simulink model "QuadSimulationSineSweepVrep"  (R2013b)
settings: Solver=ode1  StartTime=0  StopTime=10  FixedStep=0.01  MaxStep=0.06  RelTol=1e-3
model workspace (MAT data in the model file):
  Sig = Simulink.Signal
  Sig.DataType = 'auto'
  Sig.Dimensions = -1
  Sig.DimensionsMode = 'auto'
  Sig.Complexity = 'auto'
  Sig.SampleTime = -1
  Sig.SamplingMode = 'auto'
values from neighbouring files (symbols this model uses):
  IC = struct('P',(P),'Q',(Q),'R',(R),'Phi',(Phi),'The',(The),'Psi',(Psi),     'U',(U),'V',(V),'W',(W),'X',(X),'Y',(Y),'Z',(Z),'w1',(w1),'w2',(w2),'w3',(w3),'w4',(w4))    [ICgen.m]    (also in quadcopterDynamicsSFunction.m = block.DialogPrm(2).Data; quadcopterDynamicsSFunctionVrepV4.m = block.DialogPrm(2).Data; quadcopterDynamicsSFunctionVrepV5.m = block.DialogPrm(2).Data; quadcopterDynamicsSFunctionVrepV6.m = block.DialogPrm(2).Data)
  quadModel = struct('g',(g),'d',(d),'mass',(mass),'ct',(ct),'cq',(cq),     'Jx',(Jx),'Jy',(Jy),'Jz',(Jz),'Jm',(Jm),'Jb',(Jb),'Jbinv',(Jbinv),'dctcq',(dctcq),     'motor_m',(motor_m),'motor_dm',(motor_dm),'motor_h',(motor_h),'motor_r',(motor_r),     'ESC_m',(ESC_m),'ESC_a',(ESC_a),'ESC_b',(ESC_b),'ESC_ds',(ESC_ds),     'HUB_m',(HUB_m),'HUB_r',(HUB_r),'HUB_H',(HUB_H),     'arms_m',(arms_m),'arms_r',(arms_r),'arm ...(+111 chars)    [ModelGen.m]
  uart_up_p_10 = 0.9    [InitOnboardMatlab.m]
  uart_up_p_11 = 0.5    [InitOnboardMatlab.m]
  uart_up_p_12 = 0.1    [InitOnboardMatlab.m]
  uart_up_p_13 = 10    [InitOnboardMatlab.m]
  uart_up_p_14 = 50    [InitOnboardMatlab.m]
undefined symbols (not defined in the file or in its folder): DiscIntNeverNeededParam
libraries: simulink x6
Description:
  | This is a configurable quadcopter simulation.
  | This Simulink model demonstates attitude control.
  | 
  | Additional quadcopter modeling and simulation materials available at:
  | github.com/dch33/Quad-Sim
  | 
  | Copyright (C) 2014 D. Hartman, K. Landis, S. Moreno, J. Kim, M. Mehrer
  | 
  | License:
  |     This program is free software: you can redistribute it and/or modify
  |     it under the terms of the GNU LESSER GENERAL PUBLIC LICENSE as published by
  |     the Free Software Foundation, either version 3 of the License, or
  |     (at your option) any later version.
  | 
  |     This program is distributed in the hope that it will be useful,
  |     but WITHOUT ANY WARRANTY; without even the implied warranty of
  |     MERCHANTABILITY or FITNESS FOR A PARTICULAR PURPOSE.  See the
  |     GNU General Public License for more details.
  | 
  |     You should have received a copy of the GNU LESSER GENERAL PUBLIC LICENSE
  |     along with this program.  If not, see <http://www.gnu.org/licenses/>.
settings Model: ModifiedComment=Javid -- Thu Feb 04 15:27:35 2016 -- Version 1.32  Creator=David Hartman  LastModifiedBy=Javid
settings Model: ModifiedHistory=|
  | Javid -- Thu Feb 04 15:27:35 2016 -- Version 1.32
  | 
  | 
  | Javid -- Thu Feb 04 15:12:08 2016 -- Version 1.31
  | 
  | 
  | Javid -- Thu Feb 04 09:55:33 2016 -- Version 1.30
  | 
  | 
  | Javid -- Wed Feb 03 15:49:53 2016 -- Version 1.29
  | 
  | 
  | Javid -- Wed Feb 03 15:48:00 2016 -- Version 1.28
  | 
  | 
  | Javid -- Wed Feb 03 13:44:15 2016 -- Version 1.27
  | 
  | 
  | Javid -- Wed Feb 03 12:44:20 2016 -- Version 1.26
  | 
  | 
  | Javid -- Wed Feb 03 12:44:00 2016 -- Version 1.25
  | 
  | 
  | Javid -- Wed Feb 03 12:37:08 2016 -- Version 1.24
  | 
  | 
  | Javid -- Wed Feb 03 09:45:40 2016 -- Version 1.23
  | 
  | 
  | Javid -- Wed Feb 03 09:38:53 2016 -- Version 1.22
  | 
  | 
  | Javid -- Wed Feb 03 09:38:40 2016 -- Version 1.21
  | 
  | 
  | Javid -- Sat Dec 12 20:58:12 2015 -- Version 1.20
  | 
  | 
  | Javid -- Sun Nov 29 22:14:37 2015 -- Version 1.19
  | 
  | 
  | Javid -- Sun Nov 29 17:38:57 2015 -- Version 1.18
  | 
  | 
  | Javid -- Sun Nov 29 17:36:33 2015 -- Version 1.17
  | 
  | 
  | Javid -- Sun Nov 29 17:16:16 2015 -- Version 1.16
  | 
  | 
  | Javid -- Sun Nov 29 16:59:28 2015 -- Version 1.15
  | 
  | 
  | Javid -- Sun Nov 29 16:48:02 2015 -- Version 1.14
  | 
  | 
  | Javid -- Sun Nov 29 16:04:55 2015 -- Version 1.13
  | 
  | 
  | Javid -- Sat Oct 31 23:55:35 2015 -- Version 1.12
  | 
  | 
  | Javid -- Sat Oct 31 20:30:45 2015 -- Version 1.11
  | 
  | 
  | Cavid -- Mon Oct 19 16:53:56 2015 -- Version 1.10
  | 
  | 
  | Cavid -- Mon Oct 19 11:55:21 2015 -- Version 1.9
  | 
  | 
  | Cavid -- Mon Oct 19 11:50:10 2015 -- Version 1.8
  | 
  | 
  | Cavid -- Mon Oct 19 11:48:50 2015 -- Version 1.7
  | 
  | 
  | Cavid -- Mon Oct 19 11:27:32 2015 -- Version 1.6
  | 
  | 
  | davidhartman -- Fri Jun 06 23:19:51 2014 -- Version 1.5
  | 
  | 
  | davidhartman -- Fri Jun 06 22:53:10 2014 -- Version 1.3
settings SolverCC: AutoInsertRateTranBlk=on
settings DataIOCC: LimitDataPoints=off  SignalLogging=off
settings OptimizationCC: InlineParams=on
settings DebuggingCC: UniqueDataStoreMsg=warning  StateNameClashWarn=warning  StrictBusMsg=WarnOnBusTreatedAsVector

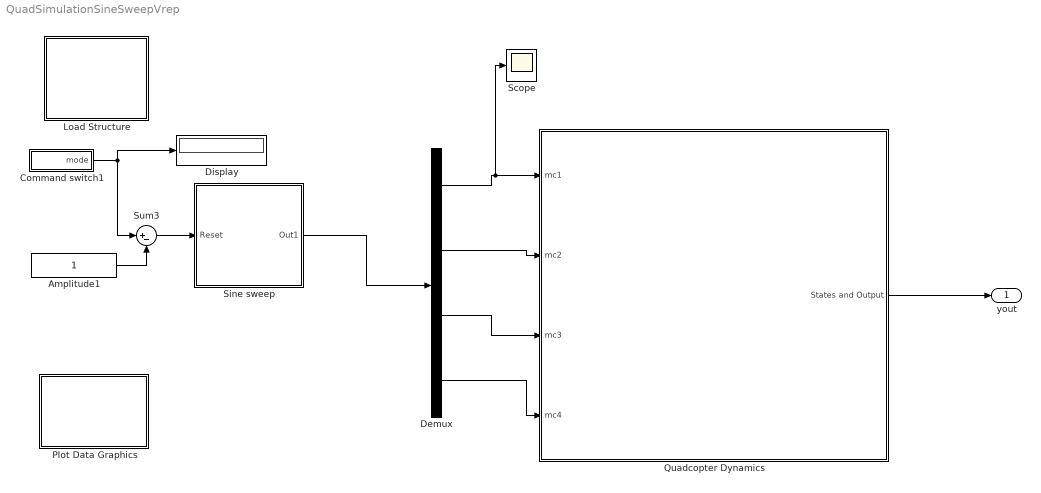
== system QuadSimulationSineSweepVrep ==
  Amplitude1 : Constant  OutMin=-2^15  OutMax=2^15-1  OutDataTypeStr=fixdt(1,32,16)
  Command switch1 : Subsystem  mask{st=[0 1.8 2.4 57 58], sa=[-0.5 -0.5 1 1 -0.5], ts=0.01, rs=on}
      mask prompts: st "Step command switching times (sec)"; sa "Step command amplitudes"; ts "Sampling time (s)"; rs "Ramp output"
  Demux : Demux
  Display : Display
  Load Structure : Subsystem
      settings: OpenFcn=|
      | uiopen('load')
      | if (exist('IC')==1 && exist('quadModel')==1)
      | set_param(bdroot, 'SimulationCommand', 'update')
      | end
      mask Display: fprintf('LOAD:\nModel and\nIC\n');
  Plot Data Graphics : Subsystem
      settings: OpenFcn=|
      | if exist('yout')
      | yout = evalin('base', 'yout');
      | tout = evalin('base', 'tout');
      | quadPlotsV5(yout, tout)
      | else
      | msgbox('Simulation must be run before data can be plotted.')
      | end
      mask Display: fprintf('Plots')
  Quadcopter Dynamics : Subsystem
  Scope : Scope
  Sine sweep : Subsystem
  Sum3 : Sum  Inputs=|+-  SaturateOnIntegerOverflow=on
  yout : Outport
  wires:
  Quadcopter Dynamics/1(States and Output) -> yout/1
  Command switch1/1(mode) -> Sum3/1, Display/1
  Amplitude1/1 -> Sum3/2
  Sum3/1 -> Sine sweep/1(Reset)
  Sine sweep/1(Out1) -> Demux/1
  Demux/1 -> Scope/1, Quadcopter Dynamics/1(mc1)
  Demux/2 -> Quadcopter Dynamics/2(mc2)
  Demux/3 -> Quadcopter Dynamics/3(mc3)
  Demux/4 -> Quadcopter Dynamics/4(mc4)

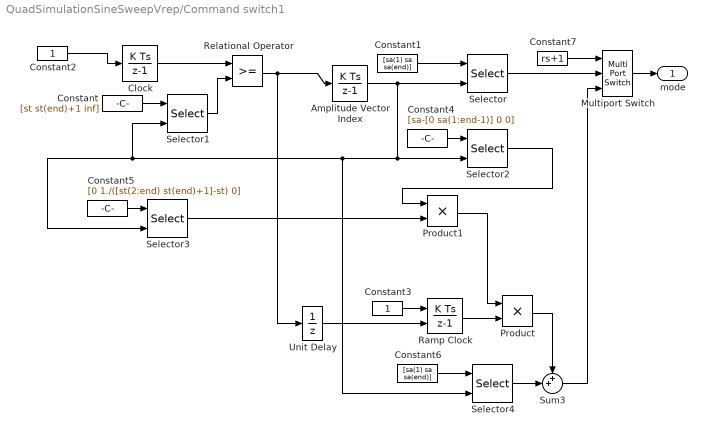
== system QuadSimulationSineSweepVrep/Command switch1 ==
  Amplitude Vector Index : DiscreteIntegrator  gainval=1/ts  InitialCondition=1  SampleTime=ts  ICPrevOutput=DiscIntNeverNeededParam  ICPrevScaledInput=DiscIntNeverNeededParam
  Clock : DiscreteIntegrator  InitialCondition=ts  SampleTime=ts  ICPrevOutput=DiscIntNeverNeededParam  ICPrevScaledInput=DiscIntNeverNeededParam
  Constant : Constant  Value=[st st(end)+1 inf]  SampleTime=ts
  Constant1 : Constant  Value=[sa(1) sa sa(end)]  SampleTime=ts
  Constant2 : Constant  SampleTime=ts
  Constant3 : Constant  SampleTime=ts
  Constant4 : Constant  Value=[sa-[0 sa(1:end-1)] 0 0]  SampleTime=ts
  Constant5 : Constant  Value=[0 1./([st(2:end) st(end)+1]-st) 0]  SampleTime=ts
  Constant6 : Constant  Value=[sa(1) sa sa(end)]  SampleTime=ts
  Constant7 : Constant  Value=rs+1  SampleTime=ts
  Multiport Switch : MultiPortSwitch  Inputs=2
  Product : Product  RndMeth=Zero
  Product1 : Product  RndMeth=Zero
  Ramp Clock : DiscreteIntegrator  ExternalReset=either  SampleTime=ts  ICPrevOutput=DiscIntNeverNeededParam  ICPrevScaledInput=DiscIntNeverNeededParam
  Relational Operator : RelationalOperator  OutDataTypeStr=uint(8)
  Selector : Selector  InputPortWidth=length(sa)+2  IndexOptions=Index vector (port)  Indices=[1 3]  OutputSizes=1
  Selector1 : Selector  InputPortWidth=length(st)+2  IndexOptions=Index vector (port)  Indices=[1 3]  OutputSizes=1
  Selector2 : Selector  InputPortWidth=length(sa)+2  IndexOptions=Index vector (port)  Indices=[1 3]  OutputSizes=1
  Selector3 : Selector  InputPortWidth=length(st)+2  IndexOptions=Index vector (port)  Indices=[1 3]  OutputSizes=1
  Selector4 : Selector  InputPortWidth=length(sa)+2  IndexOptions=Index vector (port)  Indices=[1 3]  OutputSizes=1
  Sum3 : Sum  Inputs=++|
  Unit Delay : UnitDelay  SampleTime=ts
  mode : Outport
  wires:
  Unit Delay/1 -> Ramp Clock/2
  Constant7/1 -> Multiport Switch/1
  Selector/1 -> Multiport Switch/2
  Multiport Switch/1 -> mode/1
  Sum3/1 -> Multiport Switch/3
  Selector4/1 -> Sum3/2
  Constant6/1 -> Selector4/1
  Product1/1 -> Product/1
  Selector3/1 -> Product1/2
  Constant5/1 -> Selector3/1
  Product/1 -> Sum3/1
  Ramp Clock/1 -> Product/2
  Selector2/1 -> Product1/1
  Constant4/1 -> Selector2/1
  Constant3/1 -> Ramp Clock/1
  Amplitude Vector Index/1 -> Selector/2, Selector4/2, Selector3/2, Selector1/2, Selector2/2
  Constant2/1 -> Clock/1
  Relational Operator/1 -> Unit Delay/1, Amplitude Vector Index/1
  Selector1/1 -> Relational Operator/2
  Clock/1 -> Relational Operator/1
  Constant/1 -> Selector1/1
  Constant1/1 -> Selector/1

== system QuadSimulationSineSweepVrep/Load Structure ==

== system QuadSimulationSineSweepVrep/Plot Data Graphics ==

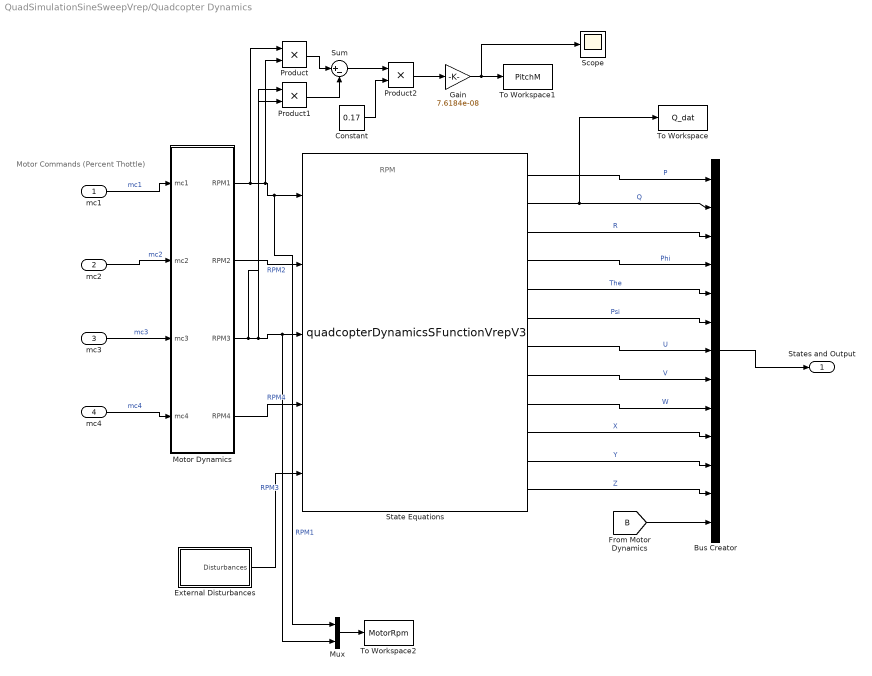
== system QuadSimulationSineSweepVrep/Quadcopter Dynamics ==
  note: Motor Commands
      | (Percent Thottle)
  note: RPM
  mc1 : Inport
  mc2 : Inport  Port=2
  mc3 : Inport  Port=3
  mc4 : Inport  Port=4
  Bus Creator : BusCreator  Inputs='P','Q','R','Phi','The','Psi','U','V','W','X','Y','Z','mc and RPM'
  Constant : Constant  Value=0.17
  External Disturbances : Subsystem
  Gain : Gain  Gain=7.6184e-08
  Motor Dynamics : Subsystem
  Mux : Mux  Inputs=2
  Product : Product
  Product1 : Product
  Product2 : Product
  Scope : Scope
      settings: YMin=-0.08  YMax=-0.0735  SaveName=ScopeData2
  State Equations : M-S-Function  FunctionName=quadcopterDynamicsSFunctionVrepV3  Parameters=quadModel, IC
      mask Display:
      | port_label('input', 1, 'RPM1')
      | port_label('input', 2, 'RPM2')
      | port_label('input', 3, 'RPM3')
      | port_label('input', 4, 'RPM4')
      | port_label('input', 5, 'Disturbances')
      | port_label('output', 1, 'P')
      | port_label('output', 2, 'Q')
      | port_label('output', 3, 'R')
      | port_label('output', 4, 'Phi')
      | port_label('output', 5, 'The')
      | port_label('output', 6, 'Psi')
      | port_label('output', 7, 'U')
      | port_label('output', 8, 'V')
      | port_label('output', 9, 'W')
      | port_label('output', 10, 'X')
      | port_label('output', 11, 'Y')
      | port_label('output', 12, 'Z')
  Sum : Sum  Inputs=|+-
  To Workspace : ToWorkspace  VariableName=Q_dat  SampleTime=-1  SaveFormat=Timeseries
  To Workspace1 : ToWorkspace  VariableName=PitchM  SampleTime=-1  SaveFormat=Timeseries
  To Workspace2 : ToWorkspace  VariableName=MotorRpm  SampleTime=-1  SaveFormat=Timeseries
  States and Output : Outport
  wires:
  [B] -> Bus Creator/13
  External Disturbances/1("Disturbances ") -> State Equations/5
  mc2/1 -> Motor Dynamics/2(mc2)  "mc2"
  mc3/1 -> Motor Dynamics/3(mc3)  "mc3"
  mc4/1 -> Motor Dynamics/4(mc4)  "mc4"
  mc1/1 -> Motor Dynamics/1(mc1)  "mc1"
  Motor Dynamics/4(RPM4) -> State Equations/4  "RPM4"
  Motor Dynamics/3(RPM3) -> Product1/1, Mux/2, State Equations/3, Product1/2  "RPM3"
  Motor Dynamics/2(RPM2) -> State Equations/2  "RPM2"
  Motor Dynamics/1(RPM1) -> Product/1, Product/2, Mux/1, State Equations/1  "RPM1"
  Bus Creator/1 -> States and Output/1
  State Equations/12 -> Bus Creator/12  "Z"
  State Equations/11 -> Bus Creator/11  "Y"
  State Equations/10 -> Bus Creator/10  "X"
  State Equations/9 -> Bus Creator/9  "W"
  State Equations/8 -> Bus Creator/8  "V"
  State Equations/7 -> Bus Creator/7  "U"
  State Equations/6 -> Bus Creator/6  "Psi"
  State Equations/5 -> Bus Creator/5  "The"
  State Equations/4 -> Bus Creator/4  "Phi"
  State Equations/3 -> Bus Creator/3  "R"
  State Equations/2 -> To Workspace/1, Bus Creator/2  "Q"
  State Equations/1 -> Bus Creator/1  "P"
  Product/1 -> Sum/1
  Product1/1 -> Sum/2
  Sum/1 -> Product2/1
  Constant/1 -> Product2/2
  Product2/1 -> Gain/1
  Gain/1 -> Scope/1, To Workspace1/1
  Mux/1 -> To Workspace2/1

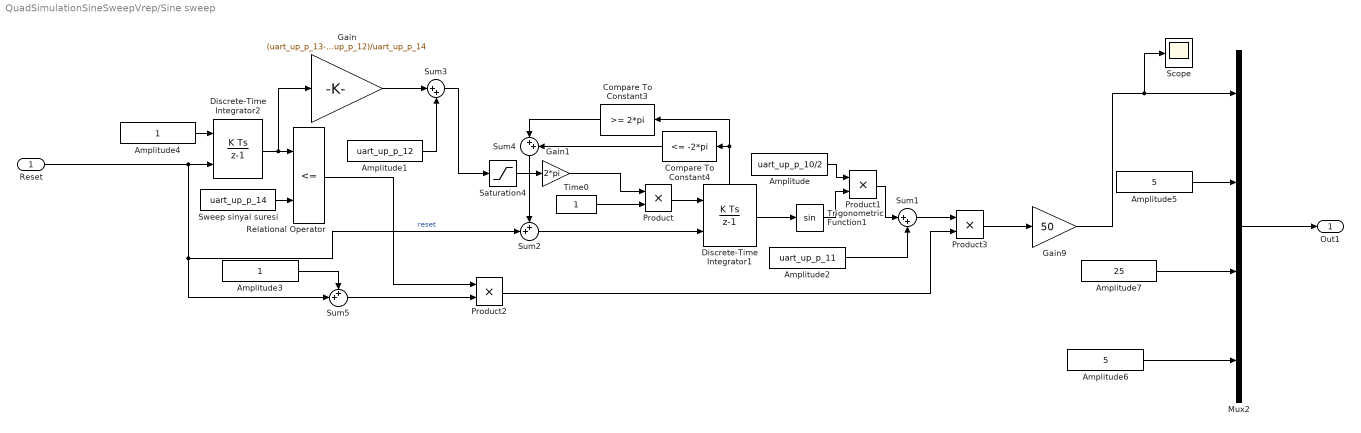
== system QuadSimulationSineSweepVrep/Sine sweep ==
  Reset : Inport
  Amplitude : Constant  Value=uart_up_p_10/2  OutMin=-2^15  OutMax=2^15-1  OutDataTypeStr=fixdt(1,32,16)
  Amplitude1 : Constant  Value=uart_up_p_12  OutMin=-2^15  OutMax=2^15-1  OutDataTypeStr=fixdt(1,32,16)
  Amplitude2 : Constant  Value=uart_up_p_11  OutMin=-2^15  OutMax=2^15-1  OutDataTypeStr=fixdt(1,32,16)
  Amplitude3 : Constant  OutMin=-2^15  OutMax=2^15-1  OutDataTypeStr=fixdt(1,32,16)
  Amplitude4 : Constant  OutMin=-2^15  OutMax=2^15-1  OutDataTypeStr=fixdt(1,32,16)
  Amplitude5 : Constant  Value=5  OutMin=-2^15  OutMax=2^15-1  OutDataTypeStr=Inherit: Inherit via back propagation
  Amplitude6 : Constant  Value=5  OutMin=-2^15  OutMax=2^15-1  OutDataTypeStr=Inherit: Inherit via back propagation
  Amplitude7 : Constant  Value=25  OutMin=-2^15  OutMax=2^15-1  OutDataTypeStr=Inherit: Inherit via back propagation
  Compare To Constant3 : simulink/Logic and Bit Operations/Compare To Constant  relop=>=  const=2*pi  OutDataTypeStr=uint8  ZeroCross=off
  Compare To Constant4 : simulink/Logic and Bit Operations/Compare To Constant  relop=<=  const=-2*pi  OutDataTypeStr=uint8  ZeroCross=off
  Discrete-Time Integrator1 : DiscreteIntegrator  ExternalReset=level  InitialConditionMode=State only (most efficient)  SampleTime=0.01  OutMax=2*pi  OutDataTypeStr=fixdt(1,32,28)  RndMeth=Zero  LimitOutput=on  UpperSaturationLimit=2*pi  LowerSaturationLimit=-2*pi  ShowStatePort=on  ICPrevOutput=DiscIntNeverNeededParam  ICPrevScaledInput=DiscIntNeverNeededParam
  Discrete-Time Integrator2 : DiscreteIntegrator  ExternalReset=level  InitialConditionMode=State only (most efficient)  SampleTime=0.01  OutDataTypeStr=fixdt(1,32,21)  RndMeth=Zero  LimitOutput=on  UpperSaturationLimit=2*pi  LowerSaturationLimit=-2*pi  ICPrevOutput=DiscIntNeverNeededParam  ICPrevScaledInput=DiscIntNeverNeededParam
  Gain : Gain  Gain=(uart_up_p_13-uart_up_p_12)/uart_up_p_14
  Gain1 : Gain  Gain=2*pi
  Gain9 : Gain  Gain=50
  Mux2 : Mux
  Product{,1..3} (4 alike) : Product
  Relational Operator : RelationalOperator  Operator=<=  OutDataTypeStr=fixdt(1,16)
  Saturation4 : Saturate  UpperLimit=32  LowerLimit=0  OutDataTypeStr=fixdt(1,16,10)  RndMeth=Zero
  Scope : Scope
      settings: YMin=55  YMax=59.5
  Sum1 : Sum  Inputs=|++  SaturateOnIntegerOverflow=on
  Sum2 : Sum  Inputs=++|  AccumDataTypeStr=int8  OutDataTypeStr=int8  SaturateOnIntegerOverflow=on
  Sum3 : Sum  Inputs=|++  SaturateOnIntegerOverflow=on
  Sum4 : Sum  Inputs=|++  AccumDataTypeStr=int8  OutDataTypeStr=int8  SaturateOnIntegerOverflow=on
  Sum5 : Sum  Inputs=++|  SaturateOnIntegerOverflow=on
  Sweep sinyal suresi : Constant  Value=uart_up_p_14  OutMin=-2^15  OutMax=2^15-1  OutDataTypeStr=fixdt(1,32,16)
  Time0 : Constant  OutDataTypeStr=fixdt(1,32,8)
  Trigonometric Function1 : Trigonometry  ApproximationMethod=CORDIC
  Out1 : Outport
  wires:
  Reset/1 -> Sum5/2, Sum2/2, Discrete-Time Integrator2/2  "reset"
  Amplitude1/1 -> Sum3/2
  Amplitude4/1 -> Discrete-Time Integrator2/1
  Sweep sinyal suresi/1 -> Relational Operator/2
  Discrete-Time Integrator2/1 -> Relational Operator/1, Gain/1
  Gain/1 -> Sum3/1
  Compare To Constant4/1 -> Sum4/2
  Compare To Constant3/1 -> Sum4/1
  Sum4/1 -> Sum2/1
  Discrete-Time Integrator1/State -> Compare To Constant3/1, Compare To Constant4/1
  Saturation4/1 -> Gain1/1
  Time0/1 -> Product/2
  Product/1 -> Discrete-Time Integrator1/1
  Discrete-Time Integrator1/1 -> Trigonometric Function1/1
  Amplitude2/1 -> Sum1/2
  Trigonometric Function1/1 -> Product1/2
  Product1/1 -> Sum1/1
  Sum3/1 -> Saturation4/1
  Gain1/1 -> Product/1
  Sum2/1 -> Discrete-Time Integrator1/2
  Amplitude/1 -> Product1/1
  Sum1/1 -> Product3/1
  Product3/1 -> Gain9/1
  Gain9/1 -> Scope/1, Mux2/1
  Relational Operator/1 -> Product2/1
  Sum5/1 -> Product2/2
  Product2/1 -> Product3/2
  Amplitude3/1 -> Sum5/1
  Mux2/1 -> Out1/1
  Amplitude7/1 -> Mux2/3
  Amplitude5/1 -> Mux2/2
  Amplitude6/1 -> Mux2/4

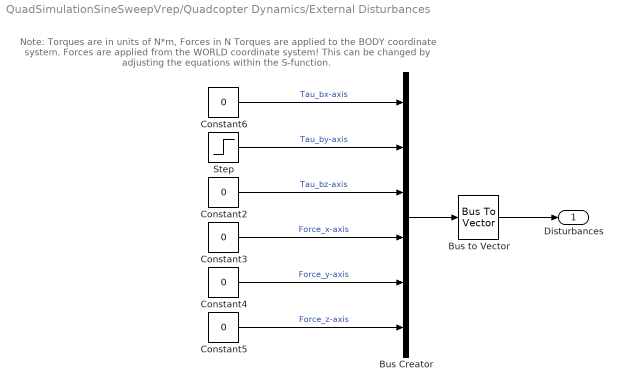
== system QuadSimulationSineSweepVrep/Quadcopter Dynamics/External Disturbances ==
  note: Note: Torques are in units of N*m, Forces in N
      | Torques are applied to the BODY coordinate system.
      | Forces are applied from the WORLD coordinate system!
      | This can be changed by adjusting the equations within the S-function.
  Bus Creator : BusCreator  Inputs=6
  Bus to Vector : BusToVector
  Constant{2..6} (5 alike) : Constant  Value=0
  Step : Step  After=0  SampleTime=0
  "Disturbances " : Outport
  wires:
  Constant5/1 -> Bus Creator/6  "Force_z-axis"
  Constant4/1 -> Bus Creator/5  "Force_y-axis"
  Constant3/1 -> Bus Creator/4  "Force_x-axis"
  Constant2/1 -> Bus Creator/3  "Tau_bz-axis"
  Step/1 -> Bus Creator/2  "Tau_by-axis"
  Constant6/1 -> Bus Creator/1  "Tau_bx-axis"
  Bus Creator/1 -> Bus to Vector/1
  Bus to Vector/1 -> "Disturbances "/1

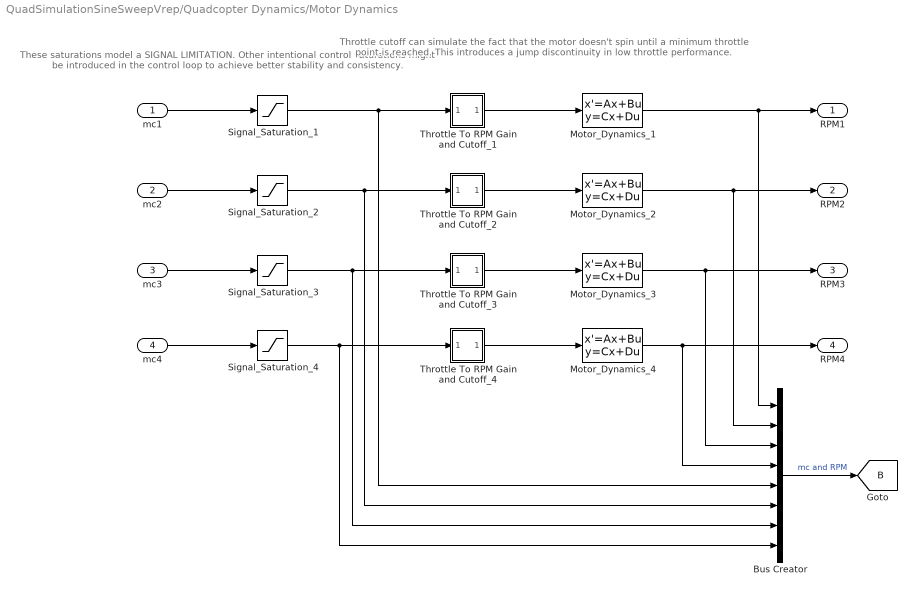
== system QuadSimulationSineSweepVrep/Quadcopter Dynamics/Motor Dynamics ==
  note: These saturations model a SIGNAL LIMITATION.
      | Other intentional control saturations might be introduced in the
      | control loop to achieve better stability and consistency.
  note: Throttle cutoff can simulate the fact that the motor doesn't
      | spin until a minimum throttle point is reached. This introduces
      | a jump discontinuity in low throttle performance.
  mc1 : Inport
  mc2 : Inport  Port=2
  mc3 : Inport  Port=3
  mc4 : Inport  Port=4
  Bus Creator : BusCreator  Inputs=8
  Motor_Dynamics_1 : StateSpace  A=-1/quadModel.T  C=1/quadModel.T  D=0  X0=IC.w1*quadModel.T
  Motor_Dynamics_2 : StateSpace  A=-1/quadModel.T  C=1/quadModel.T  D=0  X0=IC.w2*quadModel.T
  Motor_Dynamics_3 : StateSpace  A=-1/quadModel.T  C=1/quadModel.T  D=0  X0=IC.w3*quadModel.T
  Motor_Dynamics_4 : StateSpace  A=-1/quadModel.T  C=1/quadModel.T  D=0  X0=IC.w4*quadModel.T
  Signal_Saturation_{1..4} (4 alike) : Saturate  UpperLimit=100  LowerLimit=0
  Throttle To RPM Gain and Cutoff_1 : Subsystem
  Throttle To RPM Gain and Cutoff_2 : Subsystem
  Throttle To RPM Gain and Cutoff_3 : Subsystem
  Throttle To RPM Gain and Cutoff_4 : Subsystem
  RPM1 : Outport
  RPM2 : Outport  Port=2
  RPM3 : Outport  Port=3
  RPM4 : Outport  Port=4
  tag scope: B=global
  wires:
  Bus Creator/1 -> [B]  "mc and RPM"
  Motor_Dynamics_4/1 -> RPM4/1, Bus Creator/4
  Motor_Dynamics_3/1 -> RPM3/1, Bus Creator/3
  Motor_Dynamics_2/1 -> RPM2/1, Bus Creator/2
  Motor_Dynamics_1/1 -> RPM1/1, Bus Creator/1
  Throttle To RPM Gain and Cutoff_4/1(Out5) -> Motor_Dynamics_4/1
  Throttle To RPM Gain and Cutoff_3/1(Out5) -> Motor_Dynamics_3/1
  Throttle To RPM Gain and Cutoff_2/1(Out5) -> Motor_Dynamics_2/1
  Throttle To RPM Gain and Cutoff_1/1(Out5) -> Motor_Dynamics_1/1
  Signal_Saturation_4/1 -> Throttle To RPM Gain and Cutoff_4/1(In5), Bus Creator/8
  Signal_Saturation_3/1 -> Throttle To RPM Gain and Cutoff_3/1(In5), Bus Creator/7
  Signal_Saturation_2/1 -> Throttle To RPM Gain and Cutoff_2/1(In5), Bus Creator/6
  Signal_Saturation_1/1 -> Throttle To RPM Gain and Cutoff_1/1(In5), Bus Creator/5
  mc3/1 -> Signal_Saturation_3/1
  mc2/1 -> Signal_Saturation_2/1
  mc4/1 -> Signal_Saturation_4/1
  mc1/1 -> Signal_Saturation_1/1

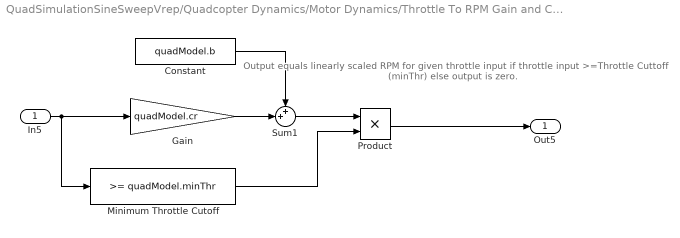
== system QuadSimulationSineSweepVrep/Quadcopter Dynamics/Motor Dynamics/Throttle To RPM Gain and Cutoff_1 ==
  note: Output equals linearly scaled RPM
      | for given throttle input if throttle input >=Throttle Cuttoff (minThr)
      | else output is zero.
  In5 : Inport
  Constant : Constant  Value=quadModel.b
  Gain : Gain  Gain=quadModel.cr
  Minimum Throttle Cutoff : simulink/Logic and Bit Operations/Compare To Constant  relop=>=  const=quadModel.minThr  OutDataTypeStr=uint8
  Product : Product
  Sum1 : Sum  Inputs=++|
  Out5 : Outport
  wires:
  Constant/1 -> Sum1/1
  Sum1/1 -> Product/1
  Gain/1 -> Sum1/2
  In5/1 -> Minimum Throttle Cutoff/1, Gain/1
  Product/1 -> Out5/1
  Minimum Throttle Cutoff/1 -> Product/2

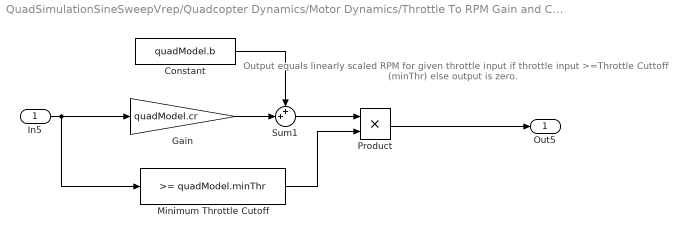
== system QuadSimulationSineSweepVrep/Quadcopter Dynamics/Motor Dynamics/Throttle To RPM Gain and Cutoff_2 ==
  note: Output equals linearly scaled RPM
      | for given throttle input if throttle input >=Throttle Cuttoff (minThr)
      | else output is zero.
  In5 : Inport
  Constant : Constant  Value=quadModel.b
  Gain : Gain  Gain=quadModel.cr
  Minimum Throttle Cutoff : simulink/Logic and Bit Operations/Compare To Constant  relop=>=  const=quadModel.minThr  OutDataTypeStr=uint8
  Product : Product
  Sum1 : Sum  Inputs=++|
  Out5 : Outport
  wires:
  Constant/1 -> Sum1/1
  Sum1/1 -> Product/1
  Gain/1 -> Sum1/2
  In5/1 -> Minimum Throttle Cutoff/1, Gain/1
  Product/1 -> Out5/1
  Minimum Throttle Cutoff/1 -> Product/2

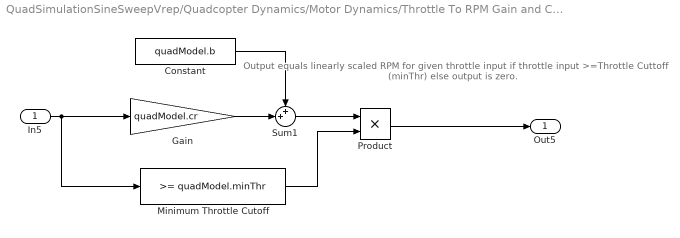
== system QuadSimulationSineSweepVrep/Quadcopter Dynamics/Motor Dynamics/Throttle To RPM Gain and Cutoff_3 ==
  note: Output equals linearly scaled RPM
      | for given throttle input if throttle input >=Throttle Cuttoff (minThr)
      | else output is zero.
  In5 : Inport
  Constant : Constant  Value=quadModel.b
  Gain : Gain  Gain=quadModel.cr
  Minimum Throttle Cutoff : simulink/Logic and Bit Operations/Compare To Constant  relop=>=  const=quadModel.minThr  OutDataTypeStr=uint8
  Product : Product
  Sum1 : Sum  Inputs=++|
  Out5 : Outport
  wires:
  Constant/1 -> Sum1/1
  Sum1/1 -> Product/1
  Gain/1 -> Sum1/2
  In5/1 -> Minimum Throttle Cutoff/1, Gain/1
  Product/1 -> Out5/1
  Minimum Throttle Cutoff/1 -> Product/2

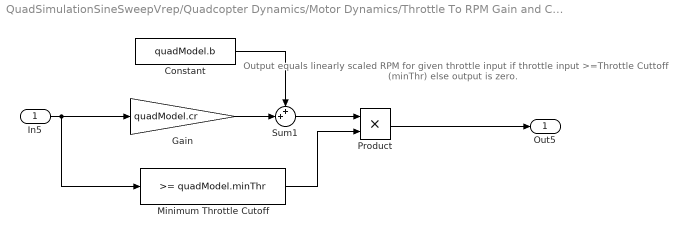
== system QuadSimulationSineSweepVrep/Quadcopter Dynamics/Motor Dynamics/Throttle To RPM Gain and Cutoff_4 ==
  note: Output equals linearly scaled RPM
      | for given throttle input if throttle input >=Throttle Cuttoff (minThr)
      | else output is zero.
  In5 : Inport
  Constant : Constant  Value=quadModel.b
  Gain : Gain  Gain=quadModel.cr
  Minimum Throttle Cutoff : simulink/Logic and Bit Operations/Compare To Constant  relop=>=  const=quadModel.minThr  OutDataTypeStr=uint8
  Product : Product
  Sum1 : Sum  Inputs=++|
  Out5 : Outport
  wires:
  Constant/1 -> Sum1/1
  Sum1/1 -> Product/1
  Gain/1 -> Sum1/2
  In5/1 -> Minimum Throttle Cutoff/1, Gain/1
  Product/1 -> Out5/1
  Minimum Throttle Cutoff/1 -> Product/2
